simulink model "fir_monit_test"  (Simulink 7.8)
settings: Solver=ode45  StartTime=0.0  StopTime=15e-4  RelTol=1e-3
undefined symbols (not defined in the file): dt_sim, xlipgetpartsetting
libraries: xbsIndex_r4 x16
settings Model: Creator=lucas.russo  LastModifiedBy=lucas.russo

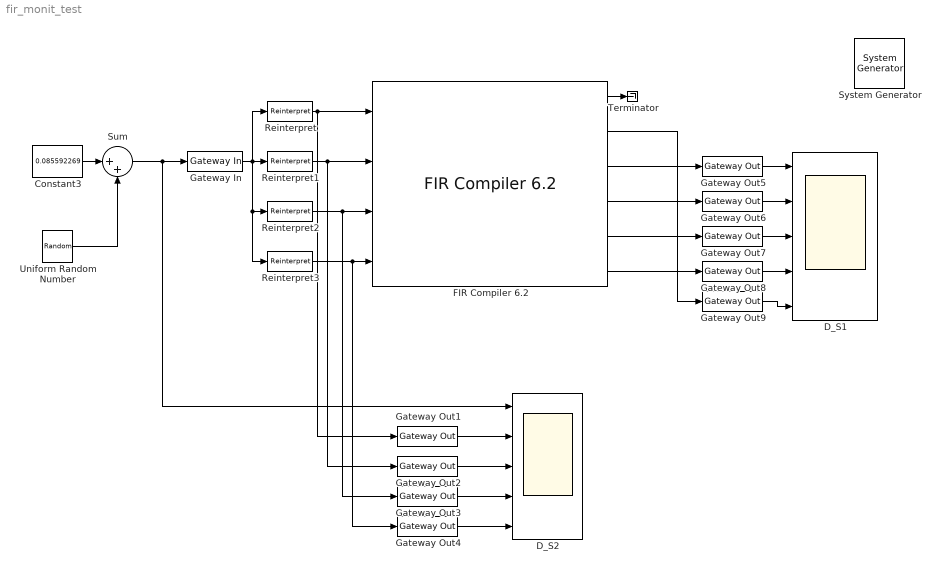
== system fir_monit_test ==
  " System Generator" : xbsIndex_r4/ System Generator  Tag=genX  xilinxfamily=virtex6  part=xc6vsx315t  speed=-3  package=ff1156  synthesis_tool=XST  clock_wrapper=Clock Enables  directory=./netlist  proj_type=Project Navigator  Synth_file=XST Defaults  Impl_file=ISE Defaults  testbench=off  simulink_period=dt_sim  sysclk_period=10  dcm_input_clock_period=10  incr_netlist=off  trim_vbits=Everywhere in SubSystem  dbl_ovrd=According to Block Masks  core_generation=According to Block Masks  run_coregen=off  deprecated_control=off  eval_field=0  block_type=sysgen
  Constant3 : Constant  Value=0.085592269  OutDataTypeStr=fixdt(1,24,23)  SampleTime=dt_sim
  D_S1 : Scope  NumInputPorts=5
      settings: TimeRange=0.0004  YMin=4.685e+010~4.685e+010~4.685e+010~4.685e+010~-5  YMax=4.725e+010~4.73e+010~4.73e+010~4.73e+010~5  SaveName=ScopeData4  MaxDataPoints=1000000  SampleInput=on
  D_S2 : Scope  NumInputPorts=5
      settings: TimeRange=0.0004  YMin=0.08535~716000~716000~0.95~-5  YMax=0.08585~720000~720000~1.05~5  MaxDataPoints=1000000  SampleInput=on
  "FIR Compiler 6.2 " : xbsIndex_r4/FIR Compiler 6.2   coefficientvector=hcfir_sec.Numerator  coefficient_sets=1  filter_type=Decimation  rate_change_type=Integer  interpolation_rate=1  decimation_rate=2  number_channels=1  ratespecification=Maximum_Possible  sampleperiod=1  hardwareoversamplingrate=1  filter_architecture=Systolic_Multiply_Accumulate  coefficient_reload=off  coefficient_sign=Signed  quantization=Integer_Coefficients  coefficient_width=16  bestprecision=off  coefficient_fractional_bits=0  coefficient_structure=Inferred  number_paths=4  output_rounding_mode=Full_Precision  output_width=34  optimization_goal=Area  data_has_tlast=Not_Required  m_data_has_tready=off  s_data_has_fifo=off  s_data_has_tuser=Not_Required  m_data_has_tuser=Not_Required  s_config_sync_mode=On_Vector  s_config_method=Single  num_reload_slots=1  has_aclken=off  has_aresetn=off  multi_column_support=Disabled  columnconfig='9'  inter_column_pipe_length=4  data_buffer_type=Automatic  coefficient_buffer_type=Automatic  input_buffer_type=Automatic  output_buffer_type=Automatic  preference_for_other_storage=Automatic  trim_axipin_name=on  passband_min=0.0  passband_max=0.5  stopband_min=0.5  stopband_max=1.0  filter_selection=1  gui_behaviour=Sysgen_GUI  data_sign=Signed  data_width=16  data_fractional_bits=0  wrapper_available=true  ip_wrap_arbitrary_binary_point=true  ip_name=FIR Compiler  ip_version=6.2  dsptool_ready=true  ipcore_usecache=true  ipcore_useipmodelcache=true  ipcore_xco_need_fpga_part=true  port_translation_map={ 'aclken' => 'en', 'aresetn' => 'rst' }  run_core_at_system_period=true  ipcore_fpga_part=xlipgetpartsetting(gcb, {'virtex6', 'xc6vlx75t', '-3', 'ff784'})  structural_sim=false  block_type=fir_compiler_v6_2
      settings: infoedit=Maximum Possible : Maximizes oversampling rate. Abstracted input handshake (no s_data_tvalid) and automatic rate propagation.<br>Hardware Oversampling Rate : Specifies oversampling rate relative to the input sample period. Abstracted input handshake (no s_data_tvalid) and automatic rate propagation.<br>Sample Period : Specifies absolute oversampling rate. No input handshake abstraction (exposes s_data_tvalid) and no rate propagation.
  Gateway In : xbsIndex_r4/Gateway In  gui_display_data_type=Fixed-point  arith_type="Signed  (2's comp)"  n_bits=24  bin_pt=23  preci_type=Single  exp_width=8  frac_width=24  quantization="Round  (unbiased: +/- Inf)"  overflow=Flag as error  period=dt_sim  dbl_ovrd=off  timing_constraint=None  locs_specified=off  LOCs={}  inherit_from_input=off  UseAsADC=off  ADCChannel='1'  hdl_port=on  block_type=gatewayin
      settings: infoedit="Gateway in block.  Converts inputs of type Simulink integer, single, double and fixed point to  Xilinx fixed-point or floating-point data type.<br><br>Hardware notes:  In hardware these blocks become top level input ports."
  Gateway Out{1..9} (9 alike) : xbsIndex_r4/Gateway Out  inherit_from_input=on  hdl_port=off  timing_constraint=None  locs_specified=off  LOCs={}  UseAsDAC=off  DACChannel='1'  block_type=gatewayout
      settings: infoedit="Gateway out block.  Converts Xilinx fixed-point or floating-point type inputs into ouputs of type Simulink integer, single, double, or fixed point.<br><br>Hardware notes:  In hardware these blocks become top level output ports or are discarded, depending on how they are configured."
  Reinterpret{,1..3} (4 alike) : xbsIndex_r4/Reinterpret  force_arith_type=on  arith_type="Signed  (2's comp)"  force_bin_pt=on  bin_pt=0  block_type=reinterpret
  Sum : Sum  Inputs=|++
  Terminator : Terminator
  Uniform Random Number : UniformRandomNumber  Minimum=-2000/(2^23)  Maximum=2000/(2^23)  Seed=6543645  SampleTime=dt_sim  VectorParams1D=off
  wires:
  Sum/1 -> Gateway In/1, D_S2/1
  Gateway In/1 -> Reinterpret2/1, Reinterpret3/1, Reinterpret/1, Reinterpret1/1
  Constant3/1 -> Sum/1
  Uniform Random Number/1 -> Sum/2
  "FIR Compiler 6.2 "/2 -> Gateway Out9/1
  "FIR Compiler 6.2 "/3 -> Gateway Out5/1
  "FIR Compiler 6.2 "/4 -> Gateway Out6/1
  "FIR Compiler 6.2 "/5 -> Gateway Out7/1
  "FIR Compiler 6.2 "/6 -> Gateway Out8/1
  "FIR Compiler 6.2 "/1 -> Terminator/1
  Gateway Out1/1 -> D_S2/2
  Gateway Out2/1 -> D_S2/3
  Gateway Out3/1 -> D_S2/4
  Gateway Out4/1 -> D_S2/5
  Gateway Out5/1 -> D_S1/1
  Gateway Out6/1 -> D_S1/2
  Gateway Out7/1 -> D_S1/3
  Gateway Out8/1 -> D_S1/4
  Gateway Out9/1 -> D_S1/5
  Reinterpret/1 -> Gateway Out1/1, "FIR Compiler 6.2 "/1
  Reinterpret1/1 -> Gateway Out2/1, "FIR Compiler 6.2 "/2
  Reinterpret2/1 -> Gateway Out3/1, "FIR Compiler 6.2 "/3
  Reinterpret3/1 -> Gateway Out4/1, "FIR Compiler 6.2 "/4
